simulink model "Gain_modelFMU"  (R2023b)
settings: Solver=FixedStepAuto  StartTime=0.0  StopTime=30  FixedStep=1  RelTol=1e-3
settings Model: PacingRate=1.050000  Creator=20181234  LastModifiedBy=20181234
settings OptimizationCC: ReuseModelBlockBuffer=off

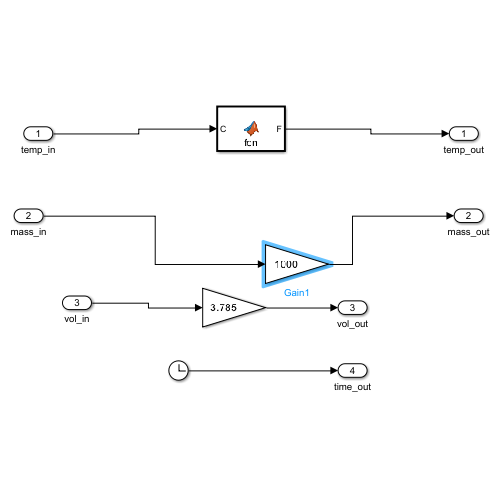
[thumbnail: Simulink's stored preview of the top-level diagram]
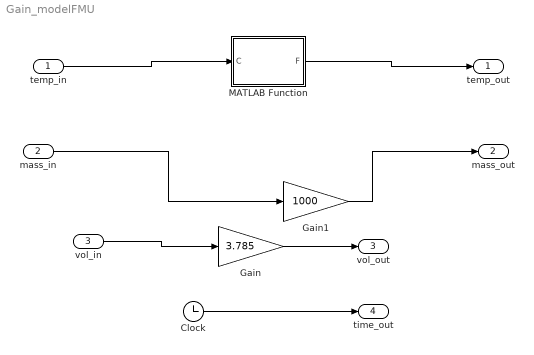
== system Gain_modelFMU ==
  temp_in : Inport
  mass_in : Inport  Port=2
  vol_in : Inport  Port=3
  Clock : Clock
  Gain : Gain  Gain=3.785
  Gain1 : Gain  Gain=1000
  MATLAB Function : MATLAB Function  TreatAsAtomicUnit=on
  temp_out : Outport
  mass_out : Outport  Port=2
  vol_out : Outport  Port=3
  time_out : Outport  Port=4
  wires:
  temp_in/1 -> MATLAB Function/1(C)
  MATLAB Function/1(F) -> temp_out/1
  Gain1/1 -> mass_out/1
  mass_in/1 -> Gain1/1
  vol_in/1 -> Gain/1
  Gain/1 -> vol_out/1
  Clock/1 -> time_out/1

== matlab function Gain_modelFMU/MATLAB Function ==
  data: C input; F output
function F = fcn(C)

F = (C*9/5)+32;
